simulink model "schem_2"  (R2024a)
settings: Solver=VariableStepAuto  StartTime=0.0  StopTime=10  RelTol=1e-3
undefined symbols (not defined in the file): k1, k2
settings Model: Creator=user  LastModifiedBy=user

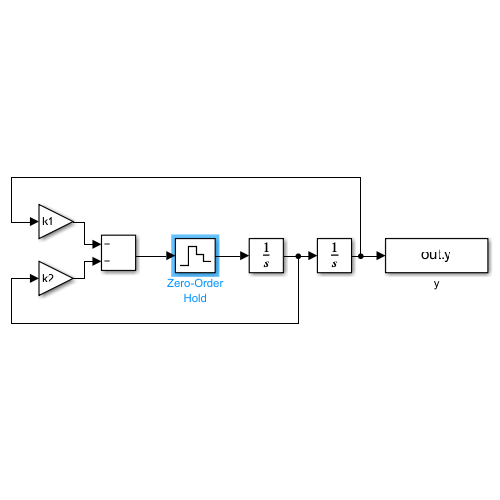
[thumbnail: Simulink's stored preview of the top-level diagram]
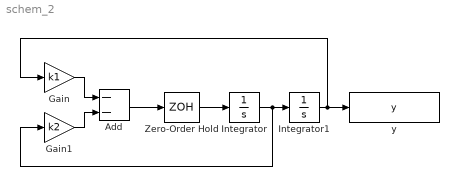
== system schem_2 ==
  Add : Sum  Inputs=--
  Gain : Gain  Gain=k1
  Gain1 : Gain  Gain=k2
  Integrator : Integrator
  Integrator1 : Integrator  InitialCondition=1
  Zero-Order Hold : ZeroOrderHold  SampleTime=0.2
  y : ToWorkspace  VariableName=y  SaveFormat=Timeseries  SampleTime=-1
  wires:
  Zero-Order Hold/1 -> Integrator/1
  Integrator/1 -> Gain1/1, Integrator1/1
  Add/1 -> Zero-Order Hold/1
  Gain1/1 -> Add/2
  Gain/1 -> Add/1
  Integrator1/1 -> Gain/1, y/1
